simulink model "hw4_4"  (R2019a)
settings: Solver=FixedStepAuto  StartTime=1  StopTime=600  FixedStep=1  RelTol=1e-3
values from neighbouring files (symbols this model uses):
  eff_motor = 0.85    [HW4.m]
  eff_transmission = 0.95    [HW4.m]
  EM_RPM = [0 1000 2000 3000 4000 5000 5300 6000 7000 8000 8500 9000 ... (24 elements, 1x24)]    [Electric_Motor_Data.mat]
  EM_torque_Nm = [260 260 260 260 260 260 260 260 260 260 260 246 ... (24 elements, 24x1)]    [Electric_Motor_Data.mat]
undefined symbols (not defined in the file or in its folder): alpha
libraries: simulink x1
settings Model: Creator=kzhai  LastModifiedBy=kzhai

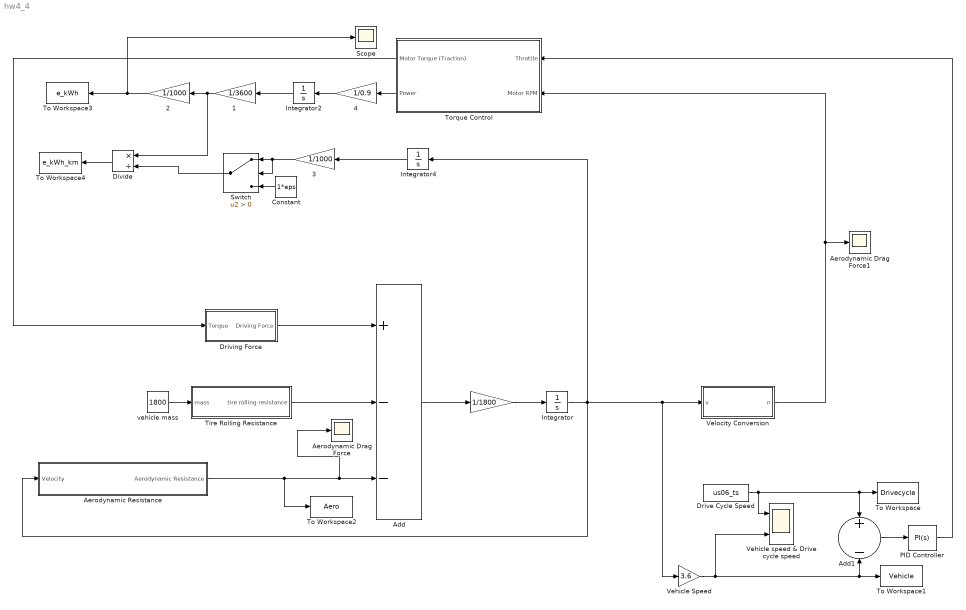
== system hw4_4 ==
  " " : Gain  Gain=1/1800
  " 1" : Gain  Gain=1/3600
  " 2" : Gain  Gain=1/1000
  " 3" : Gain  Gain=1/1000
  " 4" : Gain  Gain=1/0.9
  Add : Sum  Inputs=+--
  Add1 : Sum  Inputs=+-
  Aerodynamic Drag Force : Scope
  Aerodynamic Drag Force1 : Scope
  "Aerodynamic Resistance " : Subsystem
  Constant : Constant  Value=1*eps
  Divide : Product  Inputs=*/
  "Drive Cycle Speed " : FromWorkspace  VariableName=us06_ts  SampleTime=0
  Driving Force : Subsystem
  Integrator : Integrator
  Integrator2 : Integrator
  Integrator4 : Integrator
  PID Controller : simulink/Continuous/PID Controller  Controller=PI  Form=Parallel  TimeDomain=Continuous-time  SampleTime=-1  IntegratorMethod=Forward Euler  FilterMethod=Forward Euler  ControllerParametersSource=internal  P=1  I=1  D=0  UseFilter=on  N=100  TunerSelectOption=Transfer Function Based (PID Tuner App)  InitialConditionSource=internal  InitialConditionForIntegrator=0  InitialConditionForFilter=0  DifferentiatorICPrevScaledInput=0  ExternalReset=none  TrackingMode=off  Kt=1  LimitOutput=on  UpperSaturationLimit=1  LowerSaturationLimit=-1  LinearizeAsGain=on  AntiWindupMode=none  Kb=1  POutMin=[]  POutMax=[]  IOutMin=[]  IOutMax=[]  DOutMin=[]  DOutMax=[]  NOutMin=[]  NOutMax=[]  SumOutMin=[]  SumOutMax=[]  SaturationOutMin=[]  SaturationOutMax=[]  PParamMin=[]  PParamMax=[]  IParamMin=[]  IParamMax=[]  DParamMin=[]  DParamMax=[]  NParamMin=[]  NParamMax=[]  KbParamMin=[]  KbParamMax=[]  KtParamMin=[]  KtParamMax=[]  KbOutMin=[]  KbOutMax=[]  KtOutMin=[]  KtOutMax=[]  IntegratorOutMin=[]  IntegratorOutMax=[]  FilterOutMin=[]  FilterOutMax=[]  SumI1OutMin=[]  SumI1OutMax=[]  SumI2OutMin=[]  SumI2OutMax=[]  SumI3OutMin=[]  SumI3OutMax=[]  SumI4OutMin=[]  SumI4OutMax=[]  SumDOutMin=[]  SumDOutMax=[]  DifferentiatorOutMin=[]  DifferentiatorOutMax=[]  FilterDiffOutCoefMin=[]  FilterDiffOutCoefMax=[]  ReciprocalOutMin=[]  ReciprocalOutMax=[]  SumDenOutMin=[]  SumDenOutMax=[]  SumNumOutMin=[]  SumNumOutMax=[]  DivideOutMin=[]  DivideOutMax=[]  IntegratorContinuousStateAttributes=''  IntegratorStateMustResolveToSignalObject=off  IntegratorRTWStateStorageClass=Auto  FilterContinuousStateAttributes=''  FilterStateMustResolveToSignalObject=off  FilterRTWStateStorageClass=Auto  ParallelPVariant=InternalParameters  IdealPVariant=Disabled  IVariant=InternalParameters  DVariant=Disabled  IntegratorVariant=Continuous  SatVariant=Enabled  AWVariant=Passthrough  PCopyVariant=Disabled  TRVariant=Disabled  FdbkBlocksVariant=Forward  IdealPFdbkVariant=Disabled  SatFdbkVariant=Disabled  DerivativeFilterVariant=Disabled  NVariant=Disabled  NCopyVariant=Disabled_SignalSpec  FilterICVariant=Disabled  IntegratorICVariant=InternalICs  ExternalResetVariant=Disabled  TRSumVariant=Passthrough  SumFdbkVariant=Disabled  SumVariant=Sum_PI
  Scope : Scope
  Switch : Switch  Criteria=u2 > Threshold
  Tire Rolling Resistance : Subsystem
  To Workspace : ToWorkspace  VariableName=Drivecycle  SampleTime=-1
  To Workspace1 : ToWorkspace  VariableName=Vehicle  SampleTime=-1
  To Workspace2 : ToWorkspace  VariableName=Aero  SampleTime=-1
  To Workspace3 : ToWorkspace  VariableName=e_kWh  SampleTime=-1
  To Workspace4 : ToWorkspace  VariableName=e_kWh_km  SampleTime=-1
  "Torque Control " : Subsystem
  Vehicle Speed : Gain  Gain=3.6
  Vehicle speed & Drive cycle speed : Scope  NumInputPorts=2
  Velocity Conversion : Subsystem
  vehicle mass : Constant  Value=1800
  wires:
  Tire Rolling Resistance/1(tire rolling resistance) -> Add/2
  Driving Force/1(Driving Force) -> Add/1
  "Aerodynamic Resistance "/1(Aerodynamic Resistance) -> To Workspace2/1, Aerodynamic Drag Force/1, Add/3
  "Torque Control "/1("Motor Torque (Traction) ") -> Driving Force/1(Torque)
  Add/1 -> " "/1
  " "/1 -> Integrator/1
  Velocity Conversion/1(n) -> Aerodynamic Drag Force1/1, "Torque Control "/2(Motor RPM)
  vehicle mass/1 -> Tire Rolling Resistance/1(mass)
  Integrator/1 -> Integrator4/1, Vehicle Speed/1, Velocity Conversion/1(v), "Aerodynamic Resistance "/1(Velocity)
  "Drive Cycle Speed "/1 -> To Workspace/1, Add1/1, Vehicle speed & Drive cycle speed/1
  Vehicle Speed/1 -> To Workspace1/1, Add1/2, Vehicle speed & Drive cycle speed/2
  Add1/1 -> PID Controller/1
  PID Controller/1 -> "Torque Control "/1("Throttle ")
  Integrator2/1 -> " 1"/1
  " 1"/1 -> Divide/1, " 2"/1
  "Torque Control "/2(Power) -> " 4"/1
  Divide/1 -> To Workspace4/1
  Switch/1 -> Divide/2
  " 3"/1 -> Switch/1, Switch/2
  Constant/1 -> Switch/3
  Integrator4/1 -> " 3"/1
  " 2"/1 -> Scope/1, To Workspace3/1
  " 4"/1 -> Integrator2/1

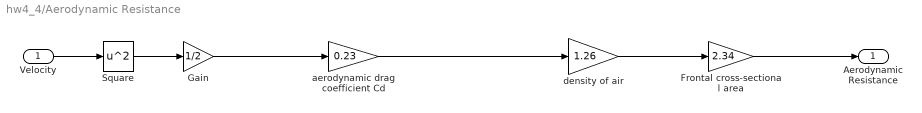
== system hw4_4/Aerodynamic Resistance  ==
  Velocity : Inport
  Frontal cross-sectional area : Gain  Gain=2.34
  Gain : Gain  Gain=1/2
  Square : Math  Operator=square  SaturateOnIntegerOverflow=on
  aerodynamic drag coefficient Cd : Gain  Gain=0.23
  density of air : Gain  Gain=1.26
  Aerodynamic Resistance : Outport
  wires:
  Frontal cross-sectional area/1 -> Aerodynamic Resistance/1
  Gain/1 -> aerodynamic drag coefficient Cd/1
  density of air/1 -> Frontal cross-sectional area/1
  Velocity/1 -> Square/1
  Square/1 -> Gain/1
  aerodynamic drag coefficient Cd/1 -> density of air/1

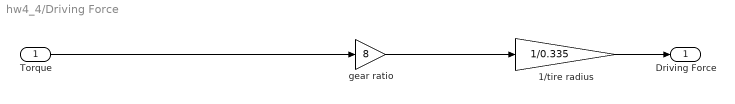
== system hw4_4/Driving Force ==
  Torque : Inport
  1/tire radius : Gain  Gain=1/0.335
  gear ratio : Gain  Gain=8
  Driving Force : Outport
  wires:
  1/tire radius/1 -> Driving Force/1
  Torque/1 -> gear ratio/1
  gear ratio/1 -> 1/tire radius/1

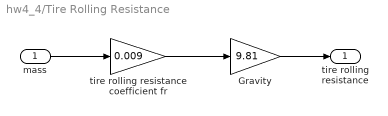
== system hw4_4/Tire Rolling Resistance ==
  mass : Inport
  Gravity : Gain  Gain=9.81
  tire rolling resistance coefficient fr : Gain  Gain=0.009
  tire rolling resistance : Outport
  wires:
  tire rolling resistance coefficient fr/1 -> Gravity/1
  Gravity/1 -> tire rolling resistance/1
  mass/1 -> tire rolling resistance coefficient fr/1

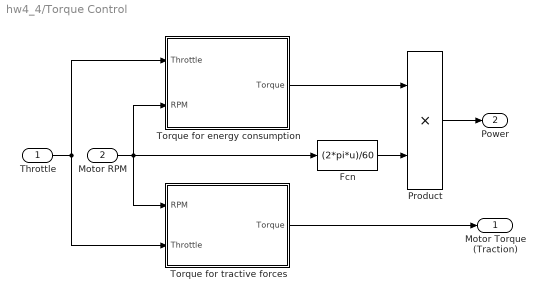
== system hw4_4/Torque Control  ==
  "Throttle " : Inport
  Motor RPM : Inport  Port=2
  Fcn : Fcn  Expr=(2*pi*u)/60
  Product : Product
  Torque for energy consumption : Subsystem
  "Torque for tractive forces " : Subsystem
  "Motor Torque (Traction) " : Outport  VectorParamsAs1DForOutWhenUnconnected=on
  Power : Outport  Port=2  VectorParamsAs1DForOutWhenUnconnected=on
  wires:
  "Torque for tractive forces "/1(Torque) -> "Motor Torque (Traction) "/1
  "Throttle "/1 -> Torque for energy consumption/1("Throttle "), "Torque for tractive forces "/2(Throttle)
  Product/1 -> Power/1
  Torque for energy consumption/1("Torque ") -> Product/1
  Motor RPM/1 -> Fcn/1, Torque for energy consumption/2(RPM), "Torque for tractive forces "/1(RPM)
  Fcn/1 -> Product/2

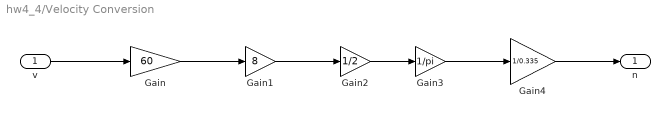
== system hw4_4/Velocity Conversion ==
  v : Inport
  Gain : Gain  Gain=60
  Gain1 : Gain  Gain=8
  Gain2 : Gain  Gain=1/2
  Gain3 : Gain  Gain=1/pi
  Gain4 : Gain  Gain=1/0.335
  n : Outport
  wires:
  Gain/1 -> Gain1/1
  Gain1/1 -> Gain2/1
  Gain2/1 -> Gain3/1
  Gain3/1 -> Gain4/1
  v/1 -> Gain/1
  Gain4/1 -> n/1

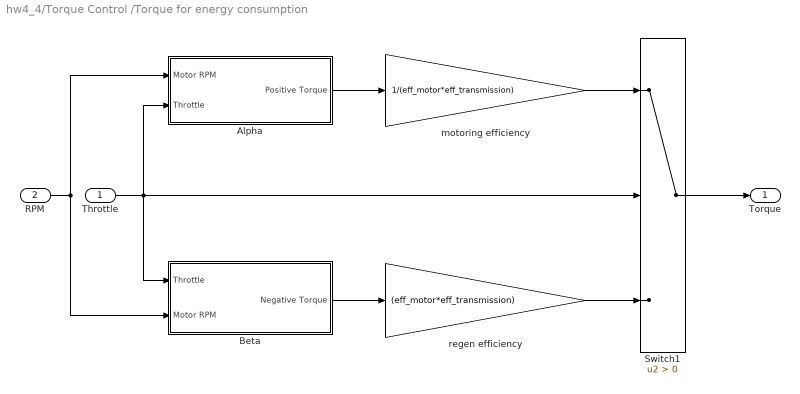
== system hw4_4/Torque Control /Torque for energy consumption ==
  "Throttle " : Inport
  RPM : Inport  Port=2
  Alpha : Subsystem
  Beta : Subsystem
  Switch1 : Switch  Criteria=u2 > Threshold
  motoring efficiency : Gain  Gain=1/(eff_motor*eff_transmission)
  regen efficiency : Gain  Gain=(eff_motor*eff_transmission)
  "Torque " : Outport  VectorParamsAs1DForOutWhenUnconnected=on
  wires:
  RPM/1 -> Alpha/1(Motor RPM), Beta/2(Motor RPM)
  "Throttle "/1 -> Beta/1(Throttle), Alpha/2(Throttle), Switch1/2
  regen efficiency/1 -> Switch1/3
  motoring efficiency/1 -> Switch1/1
  Beta/1("Negative Torque ") -> regen efficiency/1
  Alpha/1(Positive Torque) -> motoring efficiency/1
  Switch1/1 -> "Torque "/1

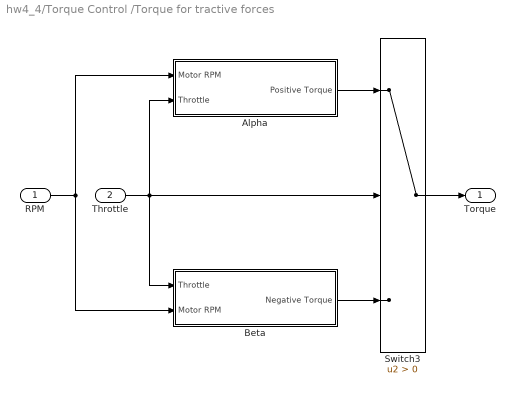
== system hw4_4/Torque Control /Torque for tractive forces  ==
  RPM : Inport
  Throttle : Inport  Port=2
  Alpha : Subsystem
  Beta : Subsystem
  Switch3 : Switch  Criteria=u2 > Threshold
  Torque : Outport  VectorParamsAs1DForOutWhenUnconnected=on
  wires:
  Throttle/1 -> Switch3/2, Beta/1("Throttle "), Alpha/2(Throttle)
  Alpha/1(Positive Torque) -> Switch3/1
  RPM/1 -> Alpha/1(Motor RPM), Beta/2(Motor RPM)
  Beta/1("Negative Torque ") -> Switch3/3
  Switch3/1 -> Torque/1

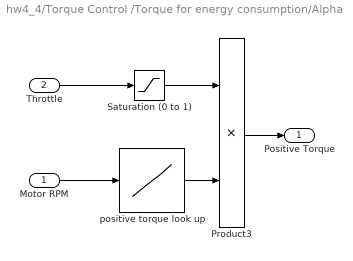
== system hw4_4/Torque Control /Torque for energy consumption/Alpha ==
  Motor RPM : Inport
  Throttle : Inport  Port=2
  Product3 : Product  RndMeth=Zero
  Saturation (0 to 1) : Saturate  UpperLimit=1  LowerLimit=0
  "positive torque look up " : Lookup_n-D  NumberOfTableDimensions=1  BreakpointsForDimension1=EM_RPM  BreakpointsForDimension2=alpha  Table=EM_torque_Nm  InternalRulePriority=Speed  RndMeth=Simplest  InputSameDT=on
  Positive Torque : Outport  VectorParamsAs1DForOutWhenUnconnected=on
  wires:
  Saturation (0 to 1)/1 -> Product3/1
  "positive torque look up "/1 -> Product3/2
  Product3/1 -> Positive Torque/1
  Throttle/1 -> Saturation (0 to 1)/1
  Motor RPM/1 -> "positive torque look up "/1

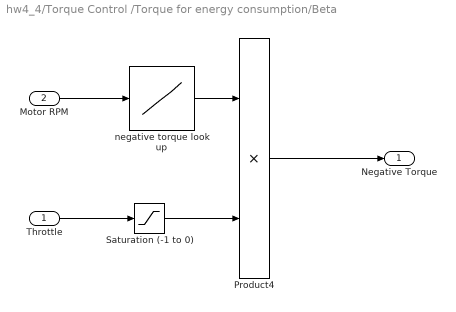
== system hw4_4/Torque Control /Torque for energy consumption/Beta ==
  Throttle : Inport
  Motor RPM : Inport  Port=2
  Product4 : Product  RndMeth=Zero
  Saturation (-1 to 0) : Saturate  UpperLimit=0  LowerLimit=-1
  "negative torque look up " : Lookup_n-D  NumberOfTableDimensions=1  BreakpointsForDimension1=EM_RPM  BreakpointsForDimension2=alpha  Table=EM_torque_Nm  InternalRulePriority=Speed  RndMeth=Simplest  InputSameDT=on
  "Negative Torque " : Outport  VectorParamsAs1DForOutWhenUnconnected=on
  wires:
  Saturation (-1 to 0)/1 -> Product4/2
  Motor RPM/1 -> "negative torque look up "/1
  "negative torque look up "/1 -> Product4/1
  Throttle/1 -> Saturation (-1 to 0)/1
  Product4/1 -> "Negative Torque "/1

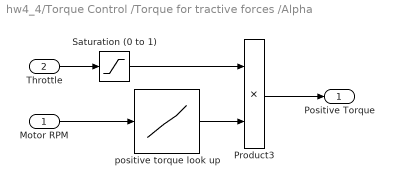
== system hw4_4/Torque Control /Torque for tractive forces /Alpha ==
  Motor RPM : Inport
  Throttle : Inport  Port=2
  Product3 : Product  RndMeth=Zero
  Saturation (0 to 1) : Saturate  UpperLimit=1  LowerLimit=0
  "positive torque look up " : Lookup_n-D  NumberOfTableDimensions=1  BreakpointsForDimension1=EM_RPM  BreakpointsForDimension2=alpha  Table=EM_torque_Nm  InternalRulePriority=Speed  RndMeth=Simplest  InputSameDT=on
  Positive Torque : Outport  VectorParamsAs1DForOutWhenUnconnected=on
  wires:
  Saturation (0 to 1)/1 -> Product3/1
  "positive torque look up "/1 -> Product3/2
  Product3/1 -> Positive Torque/1
  Throttle/1 -> Saturation (0 to 1)/1
  Motor RPM/1 -> "positive torque look up "/1

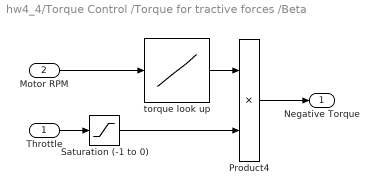
== system hw4_4/Torque Control /Torque for tractive forces /Beta ==
  "Throttle " : Inport
  Motor RPM : Inport  Port=2
  Product4 : Product  RndMeth=Zero
  Saturation (-1 to 0) : Saturate  UpperLimit=0  LowerLimit=-1
  "torque look up " : Lookup_n-D  NumberOfTableDimensions=1  BreakpointsForDimension1=EM_RPM  BreakpointsForDimension2=alpha  Table=EM_torque_Nm  InternalRulePriority=Speed  RndMeth=Simplest  InputSameDT=on
  "Negative Torque " : Outport  VectorParamsAs1DForOutWhenUnconnected=on
  wires:
  Saturation (-1 to 0)/1 -> Product4/2
  Motor RPM/1 -> "torque look up "/1
  "torque look up "/1 -> Product4/1
  "Throttle "/1 -> Saturation (-1 to 0)/1
  Product4/1 -> "Negative Torque "/1
